simulink model "Kalm_5D_2"  (Simulink 8.1)
settings: Solver=FixedStepDiscrete  StartTime=0.0  StopTime=sim_t  FixedStep=0.01  RelTol=1e-3
values from neighbouring files (symbols this model uses):
  A = zeros(15)    [init.m]
  c = 15 + lambda    [ut_weights.m]
  hparamsL = [[arms(3) arms(4), zeros(1,7)]; [m0(3,1:3) xL(1:3) s1P1L']; [m0(4,1:3) xL(4:6) s2P2L']]    [init.m]
  hparamsR = [[arms(1) arms(2), zeros(1,7)]; [m0(1,1:3) xR(1:3) s1P1R']; [m0(2,1:3) xR(4:6) s2P2R']]    [init.m]
  M0 = zeros(15,1)    [init.m]
  P0 = diag(repmat(covEps,15,1))    [init.m]
  Q = blkdiag(diag(covQ1), diag(covQ1), diag(covQ1), diag(covQ1), diag(covQ1))    [init.m]
  RL = [omega1L zeros(3,15); zeros(3,3) acc1L zeros(3,12);zeros(3,6) mag1L zeros(3,9);     zeros(3,9) omega2L zeros(3,6); zeros(3,12) acc2L zeros(3,3);zeros(3,15) mag2L]    [init.m]
  RR = [omega1R zeros(3,15); zeros(3,3) acc1R zeros(3,12);zeros(3,6) mag1R zeros(3,9);     zeros(3,9) omega2R zeros(3,6); zeros(3,12) acc2R zeros(3,3);zeros(3,15) mag2R]    [init.m]
  W = W * diag(WC) * W'    [ut_weights.m]
  WM = zeros(2*15+1,1)    [ut_weights.m]
settings Model: Creator=Lorenzo  LastModifiedBy=Alessandro
settings SolverCC: PositivePriorityOrder=on
settings DataIOCC: SaveOutput=off  SaveTime=off
settings OptimizationCC: OptimizeModelRefInitCode=on  LifeSpan=1
settings DebuggingCC: FcnCallInpInsideContextMsg=EnableAllAsWarning
settings HardwareCC: ProdHWDeviceType=Generic->Unspecified (assume 32-bit Generic)
settings ModelReferenceCC: ModelReferenceMinAlgLoopOccurrences=on
settings RTWCC: SystemTargetFile=idelink_ert.tlc  GenerateMakefile=off  TemplateMakefile=idelink_ert.tmf  Description=IDE Link ERT  ProcessScript=idelink_ert_make_rtw_hook
settings CodeAppCC: IgnoreCustomStorageClasses=off
settings TargetCC: CodeReplacementLibrary=ANSI_C  IsPILTarget=off  CompOptLevelCompliant=off  ConcurrentExecutionCompliant=on  ERTFirstTimeCompliant=on  ERTCustomFileBanners=on  SupportContinuousTime=off  SupportNonInlinedSFcns=off  EnableShiftOperators=on  ModelStepFunctionPrototypeControlCompliant=on
settings CustomProperty: DataType=string

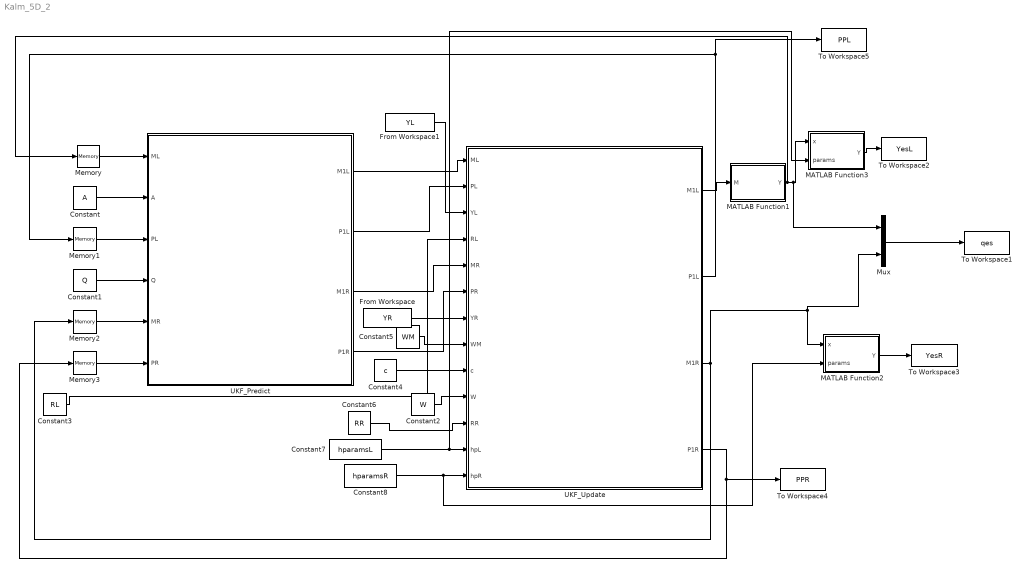
== system Kalm_5D_2 ==
  Constant : Constant  Value=A
  Constant1 : Constant  Value=Q
  Constant2 : Constant  Value=W
  Constant3 : Constant  Value=RL
  Constant4 : Constant  Value=c
  Constant5 : Constant  Value=WM
  Constant6 : Constant  Value=RR
  Constant7 : Constant  Value=hparamsL
  Constant8 : Constant  Value=hparamsR
  From Workspace : FromWorkspace  VariableName=YR  SampleTime=0.01  Interpolate=off  OutputAfterFinalValue=Holding final value
  From Workspace1 : FromWorkspace  VariableName=YL  SampleTime=0.01  Interpolate=off  OutputAfterFinalValue=Holding final value
  MATLAB Function1 : MATLAB Function  TreatAsAtomicUnit=on
  MATLAB Function2 : MATLAB Function  TreatAsAtomicUnit=on
  MATLAB Function3 : MATLAB Function  TreatAsAtomicUnit=on
  Memory : Memory  X0=M0
  Memory1 : Memory  X0=P0
  Memory2 : Memory  X0=M0
  Memory3 : Memory  X0=P0
  Mux : Mux  Inputs=2
  To Workspace1 : ToWorkspace  VariableName=qes  SampleTime=-1  SaveFormat=Structure
  To Workspace2 : ToWorkspace  VariableName=YesL  SampleTime=-1  SaveFormat=Structure
  To Workspace3 : ToWorkspace  VariableName=YesR  SampleTime=-1  SaveFormat=Structure
  To Workspace4 : ToWorkspace  VariableName=PPR  SampleTime=-1  SaveFormat=Structure
  To Workspace5 : ToWorkspace  VariableName=PPL  SampleTime=-1  SaveFormat=Structure
  UKF_Predict : Subsystem
  UKF_Update : Subsystem
  wires:
  UKF_Predict/1(M1L) -> UKF_Update/1(ML)
  UKF_Predict/2(P1L) -> UKF_Update/2(PL)
  Constant/1 -> UKF_Predict/2(A)
  Constant1/1 -> UKF_Predict/4(Q)
  Memory/1 -> UKF_Predict/1(ML)
  Constant3/1 -> UKF_Update/4(RL)
  Memory1/1 -> UKF_Predict/3(PL)
  UKF_Predict/4(P1R) -> UKF_Update/6(PR)
  UKF_Predict/3(M1R) -> UKF_Update/5(MR)
  From Workspace/1 -> UKF_Update/7(YR)
  From Workspace1/1 -> UKF_Update/3(YL)
  Memory2/1 -> UKF_Predict/5(MR)
  Memory3/1 -> UKF_Predict/6(PR)
  UKF_Update/2(P1L) -> To Workspace5/1, Memory1/1
  UKF_Update/4(P1R) -> Memory3/1, To Workspace4/1
  Mux/1 -> To Workspace1/1
  MATLAB Function3/1(Y) -> To Workspace2/1
  MATLAB Function2/1(Y) -> To Workspace3/1
  Constant5/1 -> UKF_Update/8(WM)
  Constant4/1 -> UKF_Update/9(c)
  Constant2/1 -> UKF_Update/10(W)
  UKF_Update/1(M1L) -> MATLAB Function1/1(M)
  MATLAB Function1/1(Y) -> Memory/1, Mux/1, MATLAB Function3/1(x)
  UKF_Update/3(M1R) -> Mux/2, MATLAB Function2/1(x), Memory2/1
  Constant6/1 -> UKF_Update/11(RR)
  Constant7/1 -> MATLAB Function3/2(params), UKF_Update/12(hpL)
  Constant8/1 -> MATLAB Function2/2(params), UKF_Update/13(hpR)

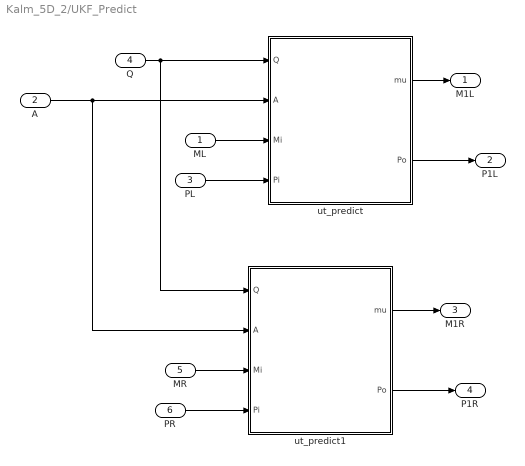
== system Kalm_5D_2/UKF_Predict ==
  ML : Inport
  A : Inport  Port=2
  PL : Inport  Port=3
  Q : Inport  Port=4
  MR : Inport  Port=5
  PR : Inport  Port=6
  ut_predict : MATLAB Function  TreatAsAtomicUnit=on
  ut_predict1 : MATLAB Function  TreatAsAtomicUnit=on
  M1L : Outport
  P1L : Outport  Port=2
  M1R : Outport  Port=3
  P1R : Outport  Port=4
  wires:
  ut_predict/1(mu) -> M1L/1
  ut_predict/2(Po) -> P1L/1
  A/1 -> ut_predict1/2(A), ut_predict/2(A)
  Q/1 -> ut_predict1/1(Q), ut_predict/1(Q)
  ML/1 -> ut_predict/3(Mi)
  PL/1 -> ut_predict/4(Pi)
  ut_predict1/1(mu) -> M1R/1
  ut_predict1/2(Po) -> P1R/1
  MR/1 -> ut_predict1/3(Mi)
  PR/1 -> ut_predict1/4(Pi)

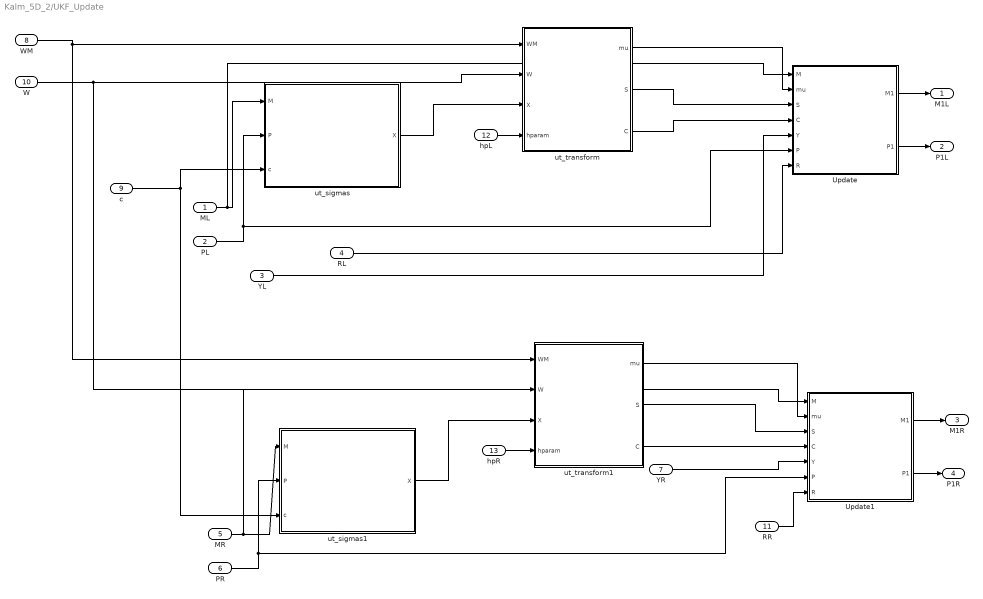
== system Kalm_5D_2/UKF_Update ==
  ML : Inport
  PL : Inport  Port=2
  YL : Inport  Port=3
  RL : Inport  Port=4
  MR : Inport  Port=5
  PR : Inport  Port=6
  YR : Inport  Port=7
  WM : Inport  Port=8
  c : Inport  Port=9
  W : Inport  Port=10
  RR : Inport  Port=11
  hpL : Inport  Port=12
  hpR : Inport  Port=13
  Update : MATLAB Function  TreatAsAtomicUnit=on
  Update1 : MATLAB Function  TreatAsAtomicUnit=on
  ut_sigmas : MATLAB Function  TreatAsAtomicUnit=on
  ut_sigmas1 : MATLAB Function  TreatAsAtomicUnit=on
  ut_transform : MATLAB Function  TreatAsAtomicUnit=on
  ut_transform1 : MATLAB Function  TreatAsAtomicUnit=on
  M1L : Outport
  P1L : Outport  Port=2
  M1R : Outport  Port=3
  P1R : Outport  Port=4
  wires:
  ut_sigmas/1(X) -> ut_transform/3(X)
  PL/1 -> ut_sigmas/2(P), Update/6(P)
  ML/1 -> ut_sigmas/1(M), Update/1(M)
  ut_transform/1(mu) -> Update/2(mu)
  ut_transform/2(S) -> Update/3(S)
  ut_transform/3(C) -> Update/4(C)
  YL/1 -> Update/5(Y)
  Update/2(P1) -> P1L/1
  RL/1 -> Update/7(R)
  Update/1(M1) -> M1L/1
  ut_sigmas1/1(X) -> ut_transform1/3(X)
  PR/1 -> ut_sigmas1/2(P), Update1/6(P)
  MR/1 -> ut_sigmas1/1(M), Update1/1(M)
  ut_transform1/1(mu) -> Update1/2(mu)
  ut_transform1/2(S) -> Update1/3(S)
  ut_transform1/3(C) -> Update1/4(C)
  YR/1 -> Update1/5(Y)
  Update1/2(P1) -> P1R/1
  Update1/1(M1) -> M1R/1
  WM/1 -> ut_transform/1(WM), ut_transform1/1(WM)
  W/1 -> ut_transform1/2(W), ut_transform/2(W)
  c/1 -> ut_sigmas1/3(c), ut_sigmas/3(c)
  RR/1 -> Update1/7(R)
  hpL/1 -> ut_transform/4(hparam)
  hpR/1 -> ut_transform1/4(hparam)

== matlab function UKF_Predict/ut_predict ==
  data: Q input double; mu output double; A input double; Po output double; Mi input double; Pi input double
function [mu,Po] = ut_predict(Q,A,Mi,Pi)
%#codegen
      
  %
  % Calculate sigma points
  %
  
%   w = {WM,WC,c};
  
  %
  % Propagate through the function
  %
  mu = A*Mi;
  Po = A*Pi*A'+Q;
end

== matlab function UKF_Update/ut_transform ==
  data: mu output double; WM input double size=[31 1]; W input double; S output double; X input double; C output double; hparam input double
function [mu,S,C] = ut_transform_h(WM,W,X, hparam)
%#codegen
      
  %
  % Calculate sigma points
  %
  
%   w = {WM,WC,c};
  
  %
  % Propagate through the function
  %
  
  Y = zeros(18,31);
  for i=1:size(X,2)
      Y(:,i) = hn_sim5DL(X(:,i), hparam);
  end
  
  
  mu = Y*WM;
  S  = Y*W*Y';
  C  = X*W*Y';
  
  
  end

== matlab function UKF_Predict/ut_predict1 ==
  data: Q input double; mu output double; A input double; Po output double; Mi input double; Pi input double
function [mu,Po] = ut_predict(Q,A,Mi,Pi)
%#codegen
      
  %
  % Calculate sigma points
  %
  
%   w = {WM,WC,c};
  
  %
  % Propagate through the function
  %
  mu = A*Mi;
  Po = A*Pi*A'+Q;
end

== matlab function UKF_Update/Update1 ==
  data: M input double; M1 output double; mu input double; S input double; C input double; Y input double; P input double; P1 output double; R input double
function [M1, P1] = update(M,mu, S, C, Y, P, R)
%#codegen
S = S+R;
K = C/S;
M1 = M+K*(Y-mu);
P1 = P-K*S*K';

== matlab function UKF_Update/ut_sigmas ==
  data: M input double size=[15 1]; X output double size=[15 31]; P input double size=[15 15]; c input double
function X = ut_sigmas(M,P,c)

%#codegen
A = chol(P)';
X = [zeros(size(M)) A -A];
X = sqrt(c)*X + repmat(M,1,size(X,2));

== matlab function UKF_Update/Update ==
  data: M input double; M1 output double; mu input double; S input double; C input double; Y input double; P input double; P1 output double; R input double
function [M1, P1] = update(M,mu, S, C, Y, P, R)
%#codegen
S = S+R;
K = C/S;
M1 = M+K*(Y-mu);
P1 = P-K*S*K';

== matlab function MATLAB Function1 ==
  data: M input double; Y output double
function Y   = thR( M )
%#codegen
Y = M;
Y(1:3:end) = atan2(sin(M(1:3:end)),cos(M(1:3:end)));

end

== matlab function MATLAB Function3 ==
  data: x input double; Y output double; params input double
function Y   = hn_sim5DL( x, params )
%#codegen
g = [0 0 -9.81]';
Z0 = [0 0 1]';
% cap2
%m02 = [17.7740   12.9559  -42.3288]';
%m01 = [16.5387   15.9820  -40.5761]';
% cap1
% m01 = [18.1780   16.3333  -39.6435]';
% m02 = [19.3934   14.7100  -41.5265]';

%Unpack params

% params first row: uarm forearm
lua = params(1,1);
lfa = params(1,2);

%[s.m0,s.qoffset,s.ry,s.rx,s.txyz];
m01 = params(2,1:3)';
m02 = params(3,1:3)';
xr = [params(2,4:6); params(3,4:6)];
p = [params(2,7:9); params(3,7:9)];

% unpack state
q = x(1:3:(5*3-2))';
dq = x(2:3:(5*3-1))';
ddq = x(3:3:(5*3))';                
    
                           
                      
%Compute parents to sensors transformations
t3 = q(3) + xr(1,1);
y1 =  xr(1,2);
x1 = xr(1,3);

S11 = [cos(t3) -sin(t3) 0 0;sin(t3) cos(t3) 0 0;0 0 1 0;0 0 0 1];
S12 = [cos(y1) 0 sin(y1) 0; 0 1 0 0;-sin(y1) 0 cos(y1) 0; 0 0 0 1];
S13 = [1 0 0 0;0 cos(x1) -sin(x1) 0;0 sin(x1) cos(x1) 0; 0 0 0 1];
S1 = S11*S12*S13;

t5 = q(5) + xr(2,1);
y2 =  xr(2,2);
x2 =  xr(2,3);

S21 = [cos(t5) -sin(t5) 0 0;sin(t5) cos(t5) 0 0;0 0 1 0;0 0 0 1];
S22 = [cos(y2) 0 sin(y2) 0; 0 1 0 0;-sin(y2) 0 cos(y2) 0; 0 0 0 1];
S23 = [1 0 0 0;0 cos(x2) -sin(x2) 0;0 sin(x2) cos(x2) 0; 0 0 0 1];
S2 = S21*S22*S23;

T = modDHL(q, lua, lfa);
T0 = [1 0 0 0;0 0 -1 0;0 1 0 0; 0 0 0 1];

%Compute joints omegas
omega1 = T(1:3,1:3)'*dq(1)*Z0;
omega2 = T(1:3,5:7)'*(omega1 + dq(2)*Z0);
omega3 = T(1:3,9:11)'*(omega2 + dq(3)*Z0);
omega4 = T(1:3,13:15)'*(omega3 + dq(4)*Z0);

%Compute joints omegadots
omegadot1 = T(1:3,1:3)'*ddq(1)*Z0;
omegadot2 = T(1:3,5:7)'*(omegadot1+cross2(dq(2)*omega1,Z0)+ddq(2)*Z0);
omegadot3 = T(1:3,9:11)'*(omegadot2+cross2(dq(3)*omega2,Z0)+ddq(3)*Z0);
omegadot4 = T(1:3,13:15)'*(omegadot3+cross2(dq(4)*omega3,Z0)+ddq(4)*Z0);

%Compute joints vdots
P1 = T(1:3,1:3)'*T(1:3,4);
vdot1 = cross2(omegadot1, P1) + cross2(omega1,cross2(omega1,P1));
P2 = T(1:3,5:7)'*T(1:3,8);
vdot2 = (cross2(omegadot2, P2)+cross2(omega2,cross2(omega2,P2))+T(1:3,5:7)'*vdot1);
P3 = T(1:3,9:11)'*T(1:3,12);
vdot3 = (cross2(omegadot3, P3)+cross2(omega3,cross2(omega3,P3))+T(1:3,9:11)'*vdot2);
P4 = T(1:3,13:15)'*T(1:3,16);
vdot4 = (cross2(omegadot4, P4)+cross2(omega4,cross2(omega4,P4))+T(1:3,13:15)'*vdot3);

%Compute sensors omegas
omegas1 = S1(1:3,1:3)'*(omega2 + dq(3)*Z0);
omegas2 = S2(1:3,1:3)'*(omega4 + dq(5)*Z0);

%Compute sensors omegadots
omegadots1 = S1(1:3,1:3)'*(omegadot2+cross2(dq(3)*omega2,Z0)+ddq(3)*Z0);
omegadots2 = S2(1:3,1:3)'*(omegadot4+cross2(dq(5)*omega4,Z0)+ddq(5)*Z0);

%Compute sensors vdots
PS1 = [p(1,:) 1]';
vdots1 = (cross2(omegadots1, PS1)+cross2(omegas1,cross2(omegas1,PS1))+S1(1:3,1:3)'*vdot2);
PS2 = [p(2,:) 1]';
vdots2 = (cross2(omegadots2, PS2)+cross2(omegas2,cross2(omegas2,PS2))+S2(1:3,1:3)'*vdot4);

Sg1 = T0(1:3,1:3)*T(1:3,1:3)*T(1:3,5:7)*S1(1:3,1:3);
Sg2 = T0(1:3,1:3)*T(1:3,1:3)*T(1:3,5:7)*T(1:3,9:11)*T(1:3,13:15)*S2(1:3,1:3);

%Compute measurement
Y = [omegas1; (vdots1+Sg1'*g)/9.81; Sg1'*m01; omegas2 ; (vdots2+Sg2'*g)/9.81; Sg2'*m02];

end


function T = modDHL(q, lua, lfa)
%#codegen

T = zeros(4,20);

dh1 = [0 pi/2 0 0 0];
dh2 = [0 pi/2 0 0 -pi/2];
dh3 = [lua 0 0 0 pi/2];
dh4 = [0 -pi/2 0 0 -pi/2];
dh5 = [0 0 lfa 0 0];

DHmatrix = [dh1;dh2;dh3;dh4;dh5];

for i=1:5
    a = DHmatrix(i,1);
    alpha = DHmatrix(i,2);
    d = DHmatrix(i,3);
    offset = DHmatrix(i,5);
    
    ct = cos(q(i) + offset);
    st = sin(q(i) + offset);
    ca = cos(alpha);
    sa = sin(alpha);
    T(1:4,(i-1)*4+1:(i-1)*4+4) = [ct -st*ca st*sa a*ct;
        st ct*ca -ct*sa a*st;
        0   sa      ca    d;
        0   0        0    1];
end


end

== matlab function UKF_Update/ut_sigmas1 ==
  data: M input double size=[15 1]; X output double size=[15 31]; P input double size=[15 15]; c input double
function X = ut_sigmas(M,P,c)

%#codegen
A = chol(P)';
X = [zeros(size(M)) A -A];
X = sqrt(c)*X + repmat(M,1,size(X,2));

== matlab function UKF_Update/ut_transform1 ==
  data: mu output double; WM input double size=[31 1]; W input double; S output double; X input double; C output double; hparam input double
function [mu,S,C] = ut_transform_h(WM,W,X, hparam)
%#codegen
      
  %
  % Calculate sigma points
  %
  
%   w = {WM,WC,c};
  
  %
  % Propagate through the function
  %
  
  Y = zeros(18,31);
  for i=1:size(X,2)
      Y(:,i) = hn_sim5DR(X(:,i), hparam);
  end
  
  
  mu = Y*WM;
  S  = Y*W*Y';
  C  = X*W*Y';
  
  
  end

== matlab function MATLAB Function2 ==
  data: x input double; Y output double; params input double
function Y   = hn_sim5DR( x, params )
%#codegen
g = [0 0 -9.81]';
Z0 = [0 0 1]';


% unpack state
q = x(1:3:(5*3-2))';
dq = x(2:3:(5*3-1))';
ddq = x(3:3:(5*3))';

%Unpack params

% params first row: uarm forearm
lua = params(1,1);
lfa = params(1,2);

%[s.m0,s.qoffset,s.ry,s.rx,s.txyz];
m01 = params(2,1:3)';
m02 = params(3,1:3)';
xr = [params(2,4:6); params(3,4:6)];
p = [params(2,7:9); params(3,7:9)];              
                     
%Compute parents to sensors transformations
%Cap2
t3 = q(3) + xr(1,1);
y1 =  xr(1,2);
x1 = xr(1,3);
          
S11 = [cos(t3) -sin(t3) 0 0;sin(t3) cos(t3) 0 0;0 0 1 0;0 0 0 1];
S12 = [cos(y1) 0 sin(y1) 0; 0 1 0 0;-sin(y1) 0 cos(y1) 0; 0 0 0 1];
S13 = [1 0 0 0;0 cos(x1) -sin(x1) 0;0 sin(x1) cos(x1) 0; 0 0 0 1];
S1 = S11*S12*S13;

%Cap2
t5 = q(5) + xr(2,1);
y2 =  xr(2,2);
x2 =  xr(2,3);

S21 = [cos(t5) -sin(t5) 0 0;sin(t5) cos(t5) 0 0;0 0 1 0;0 0 0 1];
S22 = [cos(y2) 0 sin(y2) 0; 0 1 0 0;-sin(y2) 0 cos(y2) 0; 0 0 0 1];
S23 = [1 0 0 0;0 cos(x2) -sin(x2) 0;0 sin(x2) cos(x2) 0; 0 0 0 1];
S2 = S21*S22*S23;

T = modDHR(q, lua, lfa);
T0 = [-1 0 0 0;0 0 1 0;0 1 0 0;0 0 0 1];

%Compute joints omegas
omega1 = T(1:3,1:3)'*dq(1)*Z0;
omega2 = T(1:3,5:7)'*(omega1 + dq(2)*Z0);
omega3 = T(1:3,9:11)'*(omega2 + dq(3)*Z0);
omega4 = T(1:3,13:15)'*(omega3 + dq(4)*Z0);

%Compute joints omegadots
omegadot1 = T(1:3,1:3)'*ddq(1)*Z0;
omegadot2 = T(1:3,5:7)'*(omegadot1+cross2(dq(2)*omega1,Z0)+ddq(2)*Z0);
omegadot3 = T(1:3,9:11)'*(omegadot2+cross2(dq(3)*omega2,Z0)+ddq(3)*Z0);
omegadot4 = T(1:3,13:15)'*(omegadot3+cross2(dq(4)*omega3,Z0)+ddq(4)*Z0);

%Compute joints vdots
P1 = T(1:3,1:3)'*T(1:3,4);
vdot1 = cross2(omegadot1, P1) + cross2(omega1,cross2(omega1,P1));
P2 = T(1:3,5:7)'*T(1:3,8);
vdot2 = (cross2(omegadot2, P2)+cross2(omega2,cross2(omega2,P2))+T(1:3,5:7)'*vdot1);
P3 = T(1:3,9:11)'*T(1:3,12);
vdot3 = (cross2(omegadot3, P3)+cross2(omega3,cross2(omega3,P3))+T(1:3,9:11)'*vdot2);
P4 = T(1:3,13:15)'*T(1:3,16);
vdot4 = (cross2(omegadot4, P4)+cross2(omega4,cross2(omega4,P4))+T(1:3,13:15)'*vdot3);

%Compute sensors omegas
omegas1 = S1(1:3,1:3)'*(omega2 + dq(3)*Z0);
omegas2 = S2(1:3,1:3)'*(omega4 + dq(5)*Z0);

%Compute sensors omegadots
omegadots1 = S1(1:3,1:3)'*(omegadot2+cross2(dq(3)*omega2,Z0)+ddq(3)*Z0);
omegadots2 = S2(1:3,1:3)'*(omegadot4+cross2(dq(5)*omega4,Z0)+ddq(5)*Z0);

%Compute sensors vdots
PS1 = [p(1,:) 1]';
vdots1 = (cross2(omegadots1, PS1)+cross2(omegas1,cross2(omegas1,PS1))+S1(1:3,1:3)'*vdot2);
PS2 = [p(2,:) 1]';
vdots2 = (cross2(omegadots2, PS2)+cross2(omegas2,cross2(omegas2,PS2))+S2(1:3,1:3)'*vdot4);

Sg1 = T0(1:3,1:3)*T(1:3,1:3)*T(1:3,5:7)*S1(1:3,1:3);
Sg2 = T0(1:3,1:3)*T(1:3,1:3)*T(1:3,5:7)*T(1:3,9:11)*T(1:3,13:15)*S2(1:3,1:3);

%Compute measurement
Y = [omegas1; (vdots1+Sg1'*g)/9.81; Sg1'*m01; omegas2 ; (vdots2+Sg2'*g)/9.81; Sg2'*m02];

end



function T = modDHR(q, lua, lfa)
%#codegen

T = zeros(4,20);

dh1 = [0 -pi/2 0 0 0];
dh2 = [0 -pi/2 0 0 -pi/2];
dh3 = [lua 0 0 0 pi/2];
dh4 = [0 pi/2 0 0 -pi/2];
dh5 = [0 0 -lfa 0 0];


DHmatrix = [dh1;dh2;dh3;dh4;dh5];

for i=1:5
    a = DHmatrix(i,1);
    alpha = DHmatrix(i,2);
    d = DHmatrix(i,3);
    offset = DHmatrix(i,5);
    
    ct = cos(q(i) + offset);
    st = sin(q(i) + offset);
    ca = cos(alpha);
    sa = sin(alpha);
    T(1:4,(i-1)*4+1:(i-1)*4+4) = [ct -st*ca st*sa a*ct;
        st ct*ca -ct*sa a*st;
        0   sa      ca    d;
        0   0        0    1];
end


end
